simulink model "sl_driveline"  (Simulink 7.7)
settings: Solver=ode45  StartTime=0.0  StopTime=10.0  RelTol=1e-3
undefined symbols (not defined in the file or in its folder): L
libraries: roblocks x2, simulink x1
settings Model: Creator=pic  LastModifiedBy=corkep
settings DataIOCC: LimitDataPoints=off  ReturnWorkspaceOutputs=on
settings DebuggingCC: StrictBusMsg=Warning

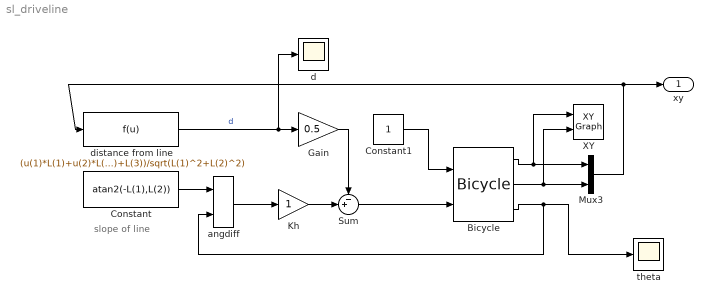
== system sl_driveline ==
  note: slope of line
  Bicycle : roblocks/Dynamics/Bicycle  SystemSampleTime=-1  accel=1  vlim=1  alim=1  L=1  x0=x0  handbrake=0
  Constant : Constant  Value=atan2(-L(1),L(2))
  Constant1 : Constant  VectorParams1D=off  SampleTime=0.02
  Gain : Gain  Gain=0.5
  Kh : Gain
  Mux3 : Mux  Inputs=2
  Sum : Sum  Inputs=-+|
  XY : simulink/Sinks/XY Graph  SystemSampleTime=-1  xmin=0  xmax=10  ymin=0  ymax=10  st=-1
  angdiff : roblocks/Trajectory/angdiff  SystemSampleTime=-1
  d : Scope
  distance from line : Fcn  Expr=(u(1)*L(1)+u(2)*L(2)+L(3))/sqrt(L(1)^2+L(2)^2)
  theta : Scope
  xy : Outport
  wires:
  Mux3/1 -> xy/1, distance from line/1
  Constant/1 -> angdiff/1
  angdiff/1 -> Kh/1
  Kh/1 -> Sum/2
  Constant1/1 -> Bicycle/1
  Sum/1 -> Bicycle/2
  distance from line/1 -> Gain/1, d/1  "d"
  Bicycle/1 -> Mux3/1, XY/1
  Bicycle/2 -> Mux3/2, XY/2
  Bicycle/3 -> theta/1, angdiff/2
  Gain/1 -> Sum/1
